simulink model "trajTest"  (R2018b)
settings: Solver=VariableStepAuto  StartTime=0.0  StopTime=1.6  FixedStep=5e-5  MaxStep=0.0002  RelTol=1e-3
libraries: model_controller x6
settings Model: Creator=Dai Luyao  LastModifiedBy=Princess
settings SFSimCC: SimUseLocalCustomCode=off
settings RTWCC: RTWUseLocalCustomCode=off
settings CodeAppCC: StateflowObjectComments=on

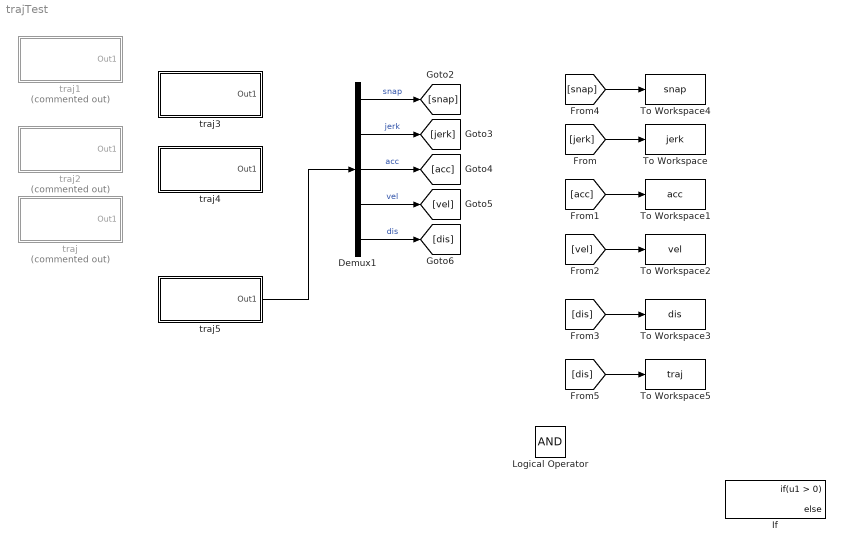
== system trajTest ==
  Demux1 : Demux  Outputs=5
  If : If
  Logical Operator : Logic  AllPortsSameDT=off  OutDataTypeStr=boolean
  To Workspace : ToWorkspace  VariableName=jerk  SaveFormat=Structure With Time  SampleTime=-1
  To Workspace1 : ToWorkspace  VariableName=acc  SaveFormat=Structure With Time  SampleTime=-1
  To Workspace2 : ToWorkspace  VariableName=vel  SaveFormat=Structure With Time  SampleTime=-1
  To Workspace3 : ToWorkspace  VariableName=dis  SaveFormat=Structure With Time  SampleTime=-1
  To Workspace4 : ToWorkspace  VariableName=snap  SaveFormat=Structure With Time  SampleTime=-1
  To Workspace5 : ToWorkspace  VariableName=traj  SampleTime=0.0002
  traj : Subsystem  Commented=on  BlockChoice=4th order traj
      link override 4th order traj: v=0.5  x=0.1  j=500
      settings: AttributesFormatString=%<BlockChoice>  TemplateBlock=model_controller/Profile Generators/traj  MemberBlocks=2th order traj,3rd order traj,4th order traj,step
  traj1 : Subsystem  Commented=on  BlockChoice=4th order traj
      link override 4th order traj: v=0.25
      settings: AttributesFormatString=%<BlockChoice>  TemplateBlock=model_controller/Profile Generators/traj  MemberBlocks=2th order traj,3rd order traj,4th order traj,step
  traj2 : Subsystem  Commented=on  BlockChoice=4th order traj
      link override 4th order traj: v=0.6  x=0.1  j=700  d=20000
      settings: AttributesFormatString=%<BlockChoice>  TemplateBlock=model_controller/Profile Generators/traj  MemberBlocks=2th order traj,3rd order traj,4th order traj,step
  traj3 : Subsystem  BlockChoice=4th order traj
      link override 3rd order traj: x=0.06  v=0.25  a=10  j=800  t0=0
      link override 4th order traj: v=0.25  x=0.05  a=10  d=64000  j=700
      settings: AttributesFormatString=%<BlockChoice>  TemplateBlock=model_controller/Profile Generators/traj  MemberBlocks=2th order traj,3rd order traj,4th order traj,step
  traj4 : Subsystem  BlockChoice=4th order traj
      link override 3rd order traj: x=0.0012  v=1  a=30  j=2000  t0=0
      link override 4th order traj: v=0.25  x=0.06  a=10  d=64000  j=800
      settings: AttributesFormatString=%<BlockChoice>  TemplateBlock=model_controller/Profile Generators/traj  MemberBlocks=2th order traj,3rd order traj,4th order traj,step
  traj5 : Subsystem  BlockChoice=4th order traj
      link override 3rd order traj: x=0.04  v=0.25  a=20  j=800  t0=0
      link override 4th order traj: v=0.2  x=0.3  a=4  d=6884  j=166  Ts=0
      settings: AttributesFormatString=%<BlockChoice>  TemplateBlock=model_controller/Profile Generators/traj  MemberBlocks=2th order traj,3rd order traj,4th order traj,step
  wires:
  Demux1/1 -> [snap]  "snap"
  Demux1/2 -> [jerk]  "jerk"
  Demux1/3 -> [acc]  "acc"
  Demux1/4 -> [vel]  "vel"
  Demux1/5 -> [dis]  "dis"
  [acc] -> To Workspace1/1
  [jerk] -> To Workspace/1
  [vel] -> To Workspace2/1
  [dis] -> To Workspace3/1
  [snap] -> To Workspace4/1
  [dis] -> To Workspace5/1
  traj5/1(Out1) -> Demux1/1

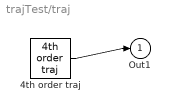
== system trajTest/traj ==
  4th order traj : model_controller/Profile Generators/4th order traj  t0=0  x=0.1  v=0.5  a=10  j=500  d=64000  Ts=0
  Out1 : Outport
  wires:
  4th order traj/1 -> Out1/1

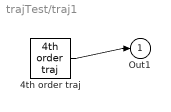
== system trajTest/traj1 ==
  4th order traj : model_controller/Profile Generators/4th order traj  t0=0  x=0.06  v=0.25  a=10  j=800  d=64000  Ts=0
  Out1 : Outport
  wires:
  4th order traj/1 -> Out1/1

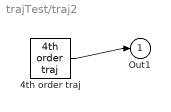
== system trajTest/traj2 ==
  4th order traj : model_controller/Profile Generators/4th order traj  t0=0  x=0.1  v=0.6  a=10  j=700  d=20000  Ts=0
  Out1 : Outport
  wires:
  4th order traj/1 -> Out1/1

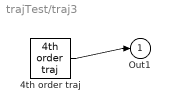
== system trajTest/traj3 ==
  4th order traj : model_controller/Profile Generators/4th order traj  t0=0  x=0.05  v=0.25  a=10  j=700  d=64000  Ts=0
  Out1 : Outport
  wires:
  4th order traj/1 -> Out1/1

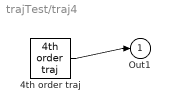
== system trajTest/traj4 ==
  4th order traj : model_controller/Profile Generators/4th order traj  t0=0  x=0.06  v=0.25  a=10  j=800  d=64000  Ts=0
  Out1 : Outport
  wires:
  4th order traj/1 -> Out1/1

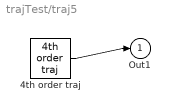
== system trajTest/traj5 ==
  4th order traj : model_controller/Profile Generators/4th order traj  t0=0  x=0.3  v=0.2  a=4  j=166  d=6884  Ts=0
  Out1 : Outport
  wires:
  4th order traj/1 -> Out1/1
